simulink model "timegaptest_gw_v2_2022b"  (R2022b)
settings: Solver=ode4  StartTime=0.0  StopTime=10.0  FixedStep=0.001  RelTol=1e-3
values from neighbouring files (symbols this model uses):
  Kdi = 0.5    [Scenario 1, 2.mat]    (also in motor_parameter_gw.m; motor_parameter_gw_v2.m = 3.9; sampleScenario_gw_v0.1.mat)
  Kdp = 1    [Scenario 1, 2.mat]    (also in motor_parameter_gw.m; motor_parameter_gw_v2.m = 4; sampleScenario_gw_v0.1.mat)
  Ki = 0.8    [Scenario 1, 2.mat]    (also in motor_parameter_gw.m; motor_parameter_gw_v2.m = 0.9; sampleScenario_gw_v0.1.mat)
  Kp = 0.5    [Scenario 1, 2.mat]    (also in motor_parameter_gw.m; motor_parameter_gw_v2.m = 0.3; sampleScenario_gw_v0.1.mat)
  Ldes = 20    [Scenario 1, 2.mat]    (also in motor_parameter_gw.m; motor_parameter_gw_v2.m; sampleScenario_gw_v0.1.mat)
  Wconst = 60    [Scenario 1, 2.mat]    (also in motor_parameter_gw.m; motor_parameter_gw_v2.m; sampleScenario_gw_v0.1.mat)
libraries: SignalEditorBlockLib x1
settings Model: Creator=현대오토1  LastModifiedBy=현대오토16
settings OptimizationCC: ReuseModelBlockBuffer=on

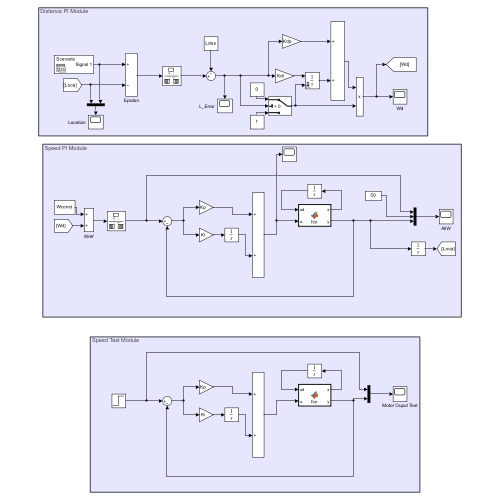
[thumbnail: Simulink's stored preview of the top-level diagram]
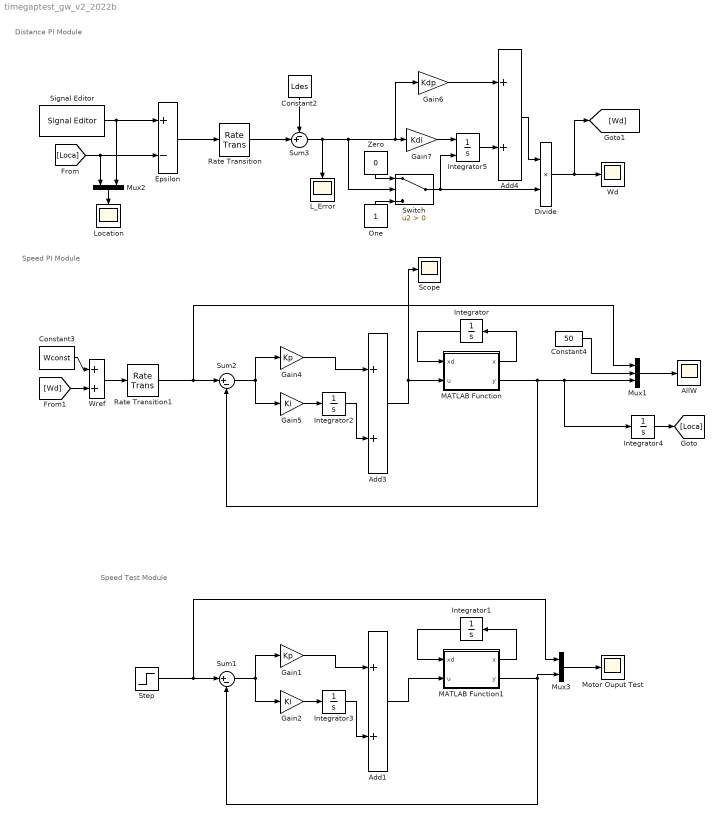
== system timegaptest_gw_v2_2022b ==
  note: Speed PI Module
  note: Distance PI Module
  note: Speed Test Module
  Add1 : Sum
  Add3 : Sum
  Add4 : Sum
  AllW : Scope
  Constant2 : Constant  Value=Ldes
  Constant3 : Constant  Value=Wconst
  Constant4 : Constant  Value=50
  Divide : Product
  Epsilon : Sum  Inputs=+-
  Gain1 : Gain  Gain=Kp
  Gain2 : Gain  Gain=Ki
  Gain4 : Gain  Gain=Kp
  Gain5 : Gain  Gain=Ki
  Gain6 : Gain  Gain=Kdp
  Gain7 : Gain  Gain=Kdi
  Integrator : Integrator  InitialCondition=[Wconst 0.4287]
  Integrator1 : Integrator
  Integrator2 : Integrator  InitialCondition=6.1
  Integrator3 : Integrator
  Integrator4 : Integrator  InitialCondition=3
  Integrator5 : Integrator  ExternalReset=either
  L_Error : Scope
  Location : Scope
  MATLAB Function : MATLAB Function  TreatAsAtomicUnit=on
  MATLAB Function1 : MATLAB Function  TreatAsAtomicUnit=on
  Motor Ouput Test : Scope
  Mux1 : Mux  Inputs=3
  Mux2 : Mux  Inputs=2
  Mux3 : Mux  Inputs=2
  One : Constant  OutDataTypeStr=Inherit: Inherit via back propagation
  Rate Transition : RateTransition  OutPortSampleTime=0.01
  Rate Transition1 : RateTransition  OutPortSampleTime=0.001
  Scope : Scope
  Signal Editor : SignalEditorBlockLib/Signal Editor  FileName=sampleScenario_gw.mat  ActiveScenario=Scenario  ActiveSignal=Signal  IsBus=off  OutputBusObjectStr=Bus: BusObject  SampleTime=0  Interpolate=off  ZeroCross=off  OutputAfterFinalValue=Setting to zero  Unit=inherit  PreserveSignalName=on
  Step : Step  After=60  SampleTime=0
  Sum1 : Sum  Inputs=|+-
  Sum2 : Sum  Inputs=|+-
  Sum3 : Sum  Inputs=-+|
  Switch : Switch  Criteria=u2 > Threshold  SaturateOnIntegerOverflow=off  InputSameDT=off
  Wd : Scope
  Wref : Sum
  Zero : Constant  Value=0  OutDataTypeStr=Inherit: Inherit via back propagation
  wires:
  Gain5/1 -> Integrator2/1
  Gain6/1 -> Add4/1
  Sum3/1 -> Switch/2, Gain7/1, Gain6/1, L_Error/1
  Gain7/1 -> Integrator5/1
  Integrator5/1 -> Add4/2
  Integrator2/1 -> Add3/2
  Sum2/1 -> Gain5/1, Gain4/1
  Gain4/1 -> Add3/1
  Mux1/1 -> AllW/1
  Integrator4/1 -> [Loca]
  [Loca] -> Mux2/1, Epsilon/2
  Signal Editor/1 -> Epsilon/1, Mux2/2
  Epsilon/1 -> Rate Transition/1
  Mux2/1 -> Location/1
  Constant4/1 -> Mux1/2
  Constant2/1 -> Sum3/1
  MATLAB Function/2(y) -> Mux1/3, Integrator4/1, Sum2/2
  MATLAB Function/1(x) -> Integrator/1
  Integrator/1 -> MATLAB Function/1(xd)
  Add3/1 -> Scope/1, MATLAB Function/2(u)
  Zero/1 -> Switch/1
  One/1 -> Switch/3
  Switch/1 -> Integrator5/2, Divide/2
  Divide/1 -> Wd/1, [Wd]
  Add4/1 -> Divide/1
  Rate Transition/1 -> Sum3/2
  Rate Transition1/1 -> Sum2/1, Mux1/1
  Constant3/1 -> Wref/1
  Wref/1 -> Rate Transition1/1
  [Wd] -> Wref/2
  Step/1 -> Mux3/1, Sum1/1
  Add1/1 -> MATLAB Function1/2(u)
  Integrator1/1 -> MATLAB Function1/1(xd)
  MATLAB Function1/1(x) -> Integrator1/1
  MATLAB Function1/2(y) -> Sum1/2, Mux3/2
  Mux3/1 -> Motor Ouput Test/1
  Gain1/1 -> Add1/1
  Sum1/1 -> Gain1/1, Gain2/1
  Integrator3/1 -> Add1/2
  Gain2/1 -> Integrator3/1

== matlab function timegaptest_gw_v2_2022b/MATLAB Function ==
  data: xd input size=2; x output size=2; u input; y output
function [x,y] = fcn(xd,u)

J = 2.09*10^(-5); %kg m 2
Kb = 0.042; %%N m A -1
Kt = 0.042;%Vrad^{-1}s^{-1}
R = 8.4; %Ω
L = 1.16; %mH
B = 0.0003; 


x= [Kt/J*xd(2)-B/J*xd(1);
    -R/L*xd(2)-Kb/L*xd(1)+1/L*u];

y=xd(1);

== matlab function timegaptest_gw_v2_2022b/MATLAB Function1 ==
  data: xd input size=2; x output size=2; u input; y output
function [x,y] = fcn(xd,u)

J = 2.09*10^(-5); %kg m 2
Kb = 0.042; %%N m A -1
Kt = 0.042;%Vrad^{-1}s^{-1}
R = 8.4; %Ω
L = 1.16; %mH
B = 0.0003; 


x= [Kt/J*xd(2)-B/J*xd(1);
    -R/L*xd(2)-Kb/L*xd(1)+1/L*u];

y=xd(1);
